simulink model "VendingMachineDesign"  (R2019b)
settings: Solver=FixedStepAuto  StartTime=0.0  StopTime=inf  RelTol=1e-3  EnableMultiTasking=on
settings Model: EnablePacing=on  Creator=Omer Eltayeb  LastModifiedBy=Omer Eltayeb
settings SolverCC: PositivePriorityOrder=on
settings OptimizationCC: EnhancedBackFolding=on  PassReuseOutputArgsAs=Individual arguments  ZeroExternalMemoryAtStartup=off  ZeroInternalMemoryAtStartup=off  MaxStackSize=64  OptimizeBlockOrder=speed  DifferentSizesBufferReuse=on  OptimizationCustomize=off  EfficientTunableParamExpr=on
settings DebuggingCC: ParameterTunabilityLossMsg=error
settings HardwareCC: ProdBitPerPointer=32  ProdBitPerSizeT=32  ProdBitPerPtrDiffT=32  ProdLargestAtomicInteger=Long  ProdLargestAtomicFloat=Double  ProdWordSize=32  ProdLongLongMode=on  ProdHWDeviceType=ARM Compatible->ARM Cortex
settings RTWCC: SystemTargetFile=ert.tlc  HardwareBoard=Raspberry Pi  TLCOptions="-aInlineSetEventsForThisBaseRateFcn=TLC_FALSE -aSuppressMultiTaskScheduler=TLC_FALSE  -aRateBasedStepFcn=0"  GenCodeOnly=on  TemplateMakefile=ert_default_tmf  GenerateReport=on  Toolchain=GNU GCC Raspberry Pi  BuildConfiguration=Faster Runs  IncludeHyperlinkInReport=on  LaunchReport=on  GenerateTraceInfo=on  GenerateTraceReport=on  GenerateTraceReportSl=on  GenerateTraceReportSf=on  GenerateTraceReportEml=on
settings CodeAppCC: ForceParamTrailComments=on  IgnoreCustomStorageClasses=off  OperatorAnnotations=on  SimulinkDataObjDesc=on  SFDataObjDesc=on  InsertBlockDesc=on
settings ERTTargetCC: SupportVariableSizeSignals=on

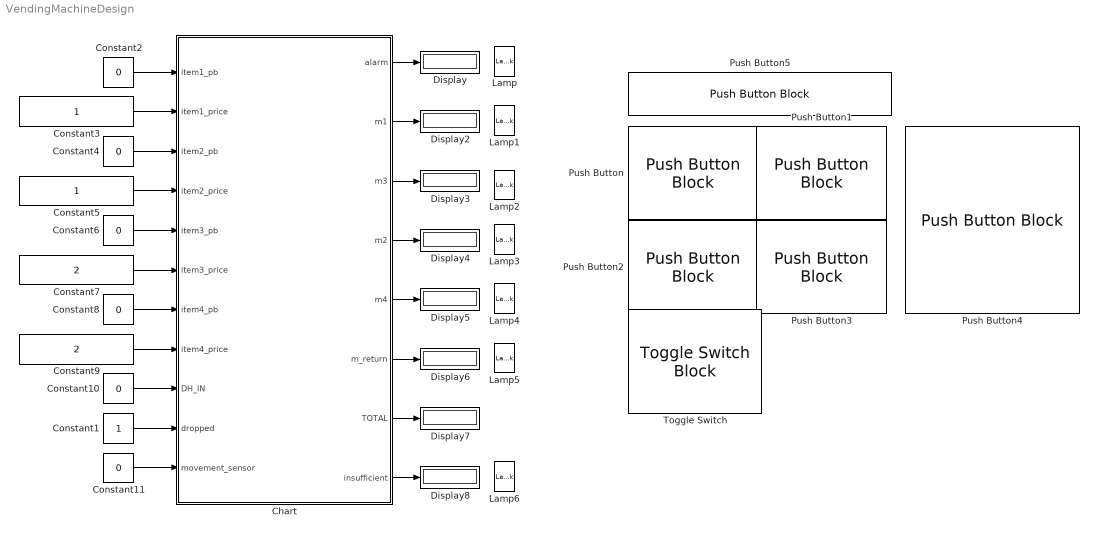
== system VendingMachineDesign ==
  Chart : Stateflow chart  BlockKeywords=__PRM__SERIALIZED__DATA__:Stateflow Chart,Stateflow Diagram  TreatAsAtomicUnit=on
  Constant1 : Constant
  Constant{2,4,6,8,10..11} (6 alike) : Constant  Value=0
  Constant3 : Constant
  Constant5 : Constant
  Constant7 : Constant  Value=2
  Constant9 : Constant  Value=2
  Display{,2..8} (8 alike) : Display
  Lamp{,1..6} (7 alike) : LampBlock  LabelPosition=Hide
  Push Button : PushButtonBlock  ButtonText=Item 1
  Push Button1 : PushButtonBlock  ButtonText=Item 2
  Push Button2 : PushButtonBlock  ButtonText=Item 3
  Push Button3 : PushButtonBlock  ButtonText=Item 4
  Push Button4 : PushButtonBlock  ButtonText=Shake Machine
  Push Button5 : PushButtonBlock  ButtonText=Insert DH
  Toggle Switch : ToggleSwitchBlock  LabelPosition=Hide
      settings: Values={{'Not Dropped', 'Dropped'}, [0 1]}
  wires:
  Constant4/1 -> Chart/3(item2_pb)
  Constant5/1 -> Chart/4(item2_price)
  Constant6/1 -> Chart/5(item3_pb)
  Constant7/1 -> Chart/6(item3_price)
  Constant8/1 -> Chart/7(item4_pb)
  Constant9/1 -> Chart/8(item4_price)
  Constant10/1 -> Chart/9(DH_IN)
  Constant2/1 -> Chart/1(item1_pb)
  Constant3/1 -> Chart/2(item1_price)
  Constant1/1 -> Chart/10(dropped)
  Constant11/1 -> Chart/11(movement_sensor)
  Chart/1(alarm) -> Display/1
  Chart/2(m1) -> Display2/1
  Chart/3(m3) -> Display3/1
  Chart/4(m2) -> Display4/1
  Chart/5(m4) -> Display5/1
  Chart/6(m_return) -> Display6/1
  Chart/7(TOTAL) -> Display7/1
  Chart/8(insufficient) -> Display8/1

== stateflow chart VendingMachineDesign/Chart ==
  state MAIN_FSM
    state IDLE
      en:
      m1 = 0;
      m2 = 0;
      m3 = 0;
      m4 = 0;
      m_return = 0;
      alarm = 0 ;
      TOTAL  = 0;
      insufficient = 0;
    state INSUFFICIENT
      en:
      m1 = 0;
      m2 = 0;
      m3 = 0;
      m4 = 0;
      insufficient = 1;
      m_return = 0;
      alarm = 0 ;
    state PAYMENT
      en:
      m1 = 0;
      m2 = 0;
      m3 = 0;
      m4 = 0;
      m_return = 0;
      alarm = 0;
      insufficient = 0;
    state ITEM_1_DROP
      en:
      m1 = 1;
      m2 = 0;
      m3 = 0;
      m4 = 0;
      m_return = 0;
      alarm = 0 ;
      TOTAL = TOTAL - item1_price;
    state ITEM_2_DROP2
      en:
      m1 = 0;
      m2 = 1;
      m3 = 0;
      m4 = 0;
      m_return = 0;
      alarm = 0 ;
      TOTAL = TOTAL - item2_price;
    state ITEM_3_DROP
      en:
      m1 = 0;
      m2 = 0;
      m3 = 1;
      m4 = 0;
      m_return = 0;
      alarm = 0 ;
      TOTAL = TOTAL - item3_price;
    state ITEM_4_DROP
      en:
      m1 = 0;
      m2 = 0;
      m3 = 0;
      m4 = 1;
      m_return = 0;
      alarm = 0 ;
      TOTAL = TOTAL - item4_price;
    state ITEM_1_WEIGHTCHECK
      en:
      m1 = 1;
      m2 = 0;
      m3 = 0;
      m4 = 0;
      m_return = 0;
      alarm = 0 ;
    state ITEM_2_WEIGHTCHECK
      en:
      m1 = 0;
      m2 = 1;
      m3 = 0;
      m4 = 0;
      m_return = 0;
      alarm = 0 ;
    state ITEM_3_WEIGHTCHECK
      en:
      m1 = 0;
      m2 = 0;
      m3 = 1;
      m4 = 0;
      m_return = 0;
      alarm = 0 ;
    state ITEM_4_WEIGHTCHECK
      en:
      m1 = 0;
      m2 = 0;
      m3 = 0;
      m4 = 1;
      m_return = 0;
      alarm = 0 ;
    state ReturnMoney
      en:
      m1 = 0;
      m2 = 0;
      m3 = 0;
      m4 = 0;
      m_return = 1;
      alarm = 0 ;
      TOTAL = TOTAL - 1;
    (default) -> IDLE
    ReturnMoney -> IDLE [order 2] : [TOTAL< 1]
    IDLE -> PAYMENT : [DH_IN == 1]/{TOTAL = TOTAL + 1;}
    INSUFFICIENT -> PAYMENT : after(2,sec)
    PAYMENT -> PAYMENT [order 5] : [DH_IN == 1]/{TOTAL = TOTAL + 1;}
    PAYMENT -> INSUFFICIENT [order 3] : [(item1_pb ==1 && TOTAL< item1_price)...
        | ||(item2_pb ==1 && TOTAL< item2_price)...
        | ||(item3_pb ==1 && TOTAL< item3_price)...
        | ||(item4_pb ==1 && TOTAL< item4_price)]
    PAYMENT -> ITEM_4_DROP [order 6] : [item4_pb ==1 &&...
        | TOTAL>= item4_price]
    PAYMENT -> ITEM_1_DROP [order 1] : [item1_pb ==1 &&...
        | TOTAL>= item1_price]
    PAYMENT -> ITEM_2_DROP2 [order 4] : [item2_pb ==1 &&...
        | TOTAL>= item2_price]
    PAYMENT -> ITEM_3_DROP [order 2] : [item3_pb ==1 &&...
        | TOTAL>= item3_price]
    ITEM_1_DROP -> ITEM_1_WEIGHTCHECK : after(3,sec)
    ITEM_2_DROP2 -> ITEM_2_WEIGHTCHECK : after(3,sec)
    ITEM_3_DROP -> ITEM_3_WEIGHTCHECK : after(3,sec)
    ITEM_4_DROP -> ITEM_4_WEIGHTCHECK : after(3,sec)
    ITEM_1_WEIGHTCHECK -> ITEM_1_WEIGHTCHECK [order 1] : after(0.5,sec)
        | [dropped~=1]
    ITEM_2_WEIGHTCHECK -> ITEM_2_WEIGHTCHECK [order 1] : after(0.5,sec)
        | [dropped~=1]
    ITEM_3_WEIGHTCHECK -> ITEM_3_WEIGHTCHECK [order 1] : after(0.5,sec)
        | [dropped~=1]
    ITEM_4_WEIGHTCHECK -> ITEM_4_WEIGHTCHECK [order 1] : after(0.5,sec)
        | [dropped~=1]
    ITEM_1_WEIGHTCHECK -> ReturnMoney [order 2] : [TOTAL>0 && dropped ~= 0]
    ITEM_2_WEIGHTCHECK -> ReturnMoney [order 2] : [TOTAL>0 && dropped ~= 0]
    ITEM_3_WEIGHTCHECK -> ReturnMoney [order 2] : [TOTAL>0 && dropped ~= 0]
    ITEM_4_WEIGHTCHECK -> ReturnMoney [order 2] : [TOTAL>0 && dropped ~= 0]
    ReturnMoney -> ReturnMoney [order 1] : after(2,sec)[TOTAL>0]
  state TURNONALARM
    en:
    m1 = 0;
    m2 = 0;
    m3 = 0;
    m4 = 0;
    m_return = 0;
    alarm = 1 ;
  (default) -> MAIN_FSM
  TURNONALARM -> IDLE [order 2] : after(10,sec)[TOTAL < 1]
  MAIN_FSM -> TURNONALARM : [movement_sensor == 1]
  TURNONALARM -> ReturnMoney [order 1] : after(10,sec)[TOTAL > 0]
  data: item1_pb input; item1_price input; item2_pb input; item2_price input; item3_pb input; item3_price input; item4_pb input; item4_price input; alarm output; m1 output; m3 output; m2 output; m4 output; m_return output; DH_IN input; dropped input; TOTAL output; insufficient output; movement_sensor input
